simulink model "Nielin_stepinfo"  (R2017a)
settings: Solver=VariableStepAuto  StartTime=0.0  StopTime=10.0  RelTol=1e-3
values from neighbouring files (symbols this model uses):
  A = pi*R1*R1    (= 10.9999393421)    [Lab2.m]    (also in ModelDataNonlinear.m)
  B = (pi*R2*R2)/(3*H2*H2)    (= 0.00337009933323)    [Lab2.m]    (also in Lab8.m = deltah20max / k; Lab9.m = 0.4; ModelDataNonlinear.m)
  C1 = 1.372    [Lab2.m]    (also in ModelDataNonlinear.m)
  C2 = 0.332756    [Lab2.m]    (also in ModelDataNonlinear.m)
  h10 = (q10/C1).^2    [Lab2.m]    (also in ModelDataNonlinear.m)
  h20 = h2max/2    (= 8)    [Lab2.m]    (also in ModelDataNonlinear.m)
  Kr = 0.14    [Lab3.m]    (also in Lab4.m = kr * (1 + 1/(Ti*s) + (Td*s)/(Tf*s+1)); Lab5.m = minreal(kr_gwiazdka * ((1 + s*Ta) * (1 + s*Tc)) / (s*(1 + s*; Lab6.m = 0.2647; Lab7.m = (1 / K) * (Gm / (1 - Gm)))
  T3 = 8    [Lab1.m]    (also in Lab3.m = 0.5*T1; Lab4.m = 0.5 * T1; ModelData.m = min(T1, T2) / 2)
settings Model: Creator=ishiguro  LastModifiedBy=ishiguro

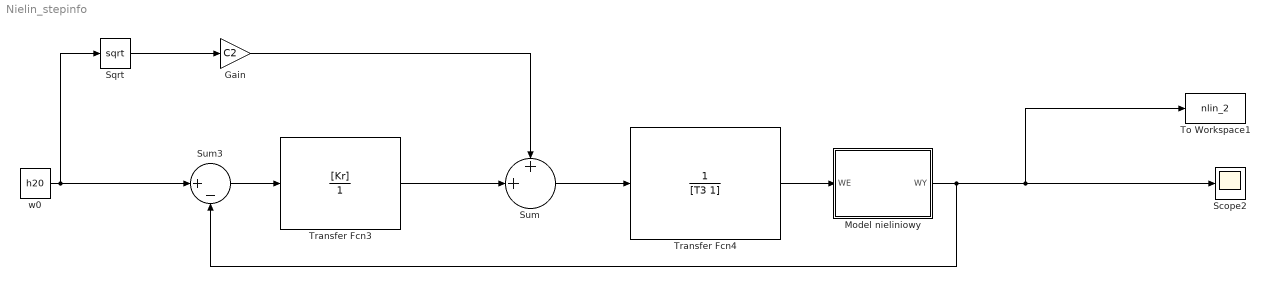
== system Nielin_stepinfo ==
  Gain : Gain  Gain=C2
  Model nieliniowy : Subsystem
  Scope2 : Scope
  Sqrt : Sqrt  SaturateOnIntegerOverflow=on
  Sum : Sum  Inputs=++|
  Sum3 : Sum  Inputs=|+-
  To Workspace1 : ToWorkspace  VariableName=nlin_2  SampleTime=-1
  Transfer Fcn3 : TransferFcn  Numerator=[Kr]  Denominator=[1]
  Transfer Fcn4 : TransferFcn  Denominator=[T3 1]
  w0 : Constant  Value=h20
  wires:
  Sqrt/1 -> Gain/1
  Transfer Fcn3/1 -> Sum/2
  Model nieliniowy/1(WY) -> Sum3/2, To Workspace1/1, Scope2/1
  Gain/1 -> Sum/1
  Sum/1 -> Transfer Fcn4/1
  w0/1 -> Sum3/1, Sqrt/1
  Transfer Fcn4/1 -> Model nieliniowy/1(WE)
  Sum3/1 -> Transfer Fcn3/1

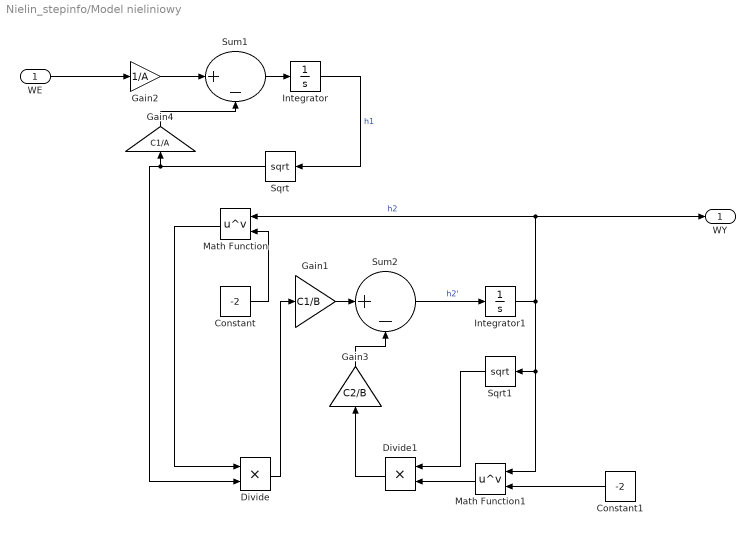
== system Nielin_stepinfo/Model nieliniowy ==
  WE : Inport
  Constant : Constant  Value=-2
  Constant1 : Constant  Value=-2
  Divide : Product  Inputs=**
  Divide1 : Product  Inputs=**
  Gain1 : Gain  Gain=C1/B
  Gain2 : Gain  Gain=1/A
  Gain3 : Gain  Gain=C2/B
  Gain4 : Gain  Gain=C1/A
  Integrator : Integrator  InitialCondition=h10
  Integrator1 : Integrator  InitialCondition=h20
  Math Function : Math  Operator=pow  SaturateOnIntegerOverflow=on
  Math Function1 : Math  Operator=pow  SaturateOnIntegerOverflow=on
  Sqrt : Sqrt  SaturateOnIntegerOverflow=on
  Sqrt1 : Sqrt  SaturateOnIntegerOverflow=on
  Sum1 : Sum  Inputs=|+-
  Sum2 : Sum  Inputs=|+-
  WY : Outport
  wires:
  Sum1/1 -> Integrator/1
  Sqrt1/1 -> Divide1/1
  Gain4/1 -> Sum1/2
  Integrator1/1 -> Math Function/1, WY/1, Math Function1/1, Sqrt1/1  "h2"
  Sqrt/1 -> Divide/2, Gain4/1
  Gain3/1 -> Sum2/2
  Sum2/1 -> Integrator1/1  "h2'"
  Divide1/1 -> Gain3/1
  Integrator/1 -> Sqrt/1  "h1"
  Gain1/1 -> Sum2/1
  Divide/1 -> Gain1/1
  Gain2/1 -> Sum1/1
  WE/1 -> Gain2/1
  Constant/1 -> Math Function/2
  Math Function/1 -> Divide/1
  Math Function1/1 -> Divide1/2
  Constant1/1 -> Math Function1/2
